simulink model "SIMPLEAC"  (R2020b)
settings: Solver=VariableStepAuto  StartTime=0.0  StopTime=7200  RelTol=1e-3
libraries: simulink x3
settings Model: Creator=99003197  LastModifiedBy=99003181
settings DebuggingCC: ArithmeticOperatorsInVariantConditions=warning
settings SFSimCC: CustomCodeUndefinedFunction=UseInterfaceOnly

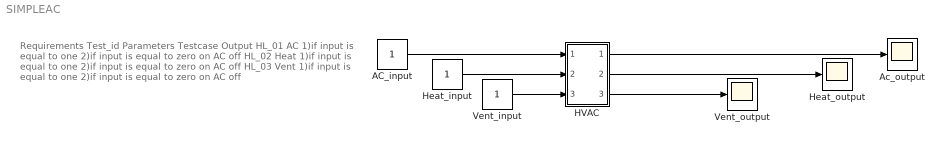
== system SIMPLEAC ==
  note: Requirements
      | Test_id
      | Parameters
      | Testcase
      | Output
      |
      | HL_01
      | AC
      | 1)if input is equal to one
      | 2)if input is equal to zero
      |
      | on
      |
      | AC off
      |
      | HL_02
      | Heat
      | 1)if input is equal to one
      | 2)if input is equal to zero
      | on
      |
      | AC off
      |
      | HL_03
      | Vent
      | 1)if input is equal to one
      | 2)if input is equal to zero
      | on
      |
      | AC off
  AC_input : Constant
  Ac_output : Scope
  HVAC : Subsystem
  Heat_input : Constant
  Heat_output : Scope
  Vent_input : Constant
  Vent_output : Scope
  wires:
  Heat_input/1 -> HVAC/2(Input1)
  AC_input/1 -> HVAC/1(Input)
  HVAC/1(Output) -> Ac_output/1
  Vent_input/1 -> HVAC/3(Input2)
  HVAC/2(Output1) -> Heat_output/1
  HVAC/3(Output2) -> Vent_output/1

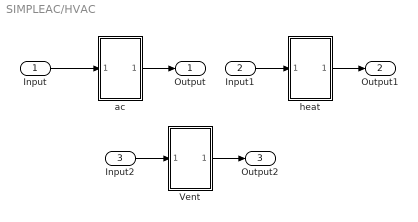
== system SIMPLEAC/HVAC ==
  Input : Inport
  Input1 : Inport  Port=2
  Input2 : Inport  Port=3
  Vent : Subsystem
  ac : Subsystem
  heat : Subsystem
  Output : Outport
  Output1 : Outport  Port=2
  Output2 : Outport  Port=3
  wires:
  Input/1 -> ac/1(Input)
  Input1/1 -> heat/1(Input)
  ac/1(Output) -> Output/1
  heat/1(Output) -> Output1/1
  Input2/1 -> Vent/1(Input)
  Vent/1(Output) -> Output2/1

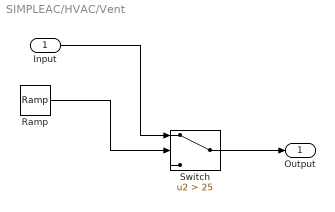
== system SIMPLEAC/HVAC/Vent ==
  Input : Inport
  Ramp : simulink/Sources/Ramp  slope=-0.0069  start=0  InitialOutput=50
  Switch : Switch  Criteria=u2 > Threshold  Threshold=25
  Output : Outport
  wires:
  Ramp/1 -> Switch/2
  Input/1 -> Switch/1
  Switch/1 -> Output/1

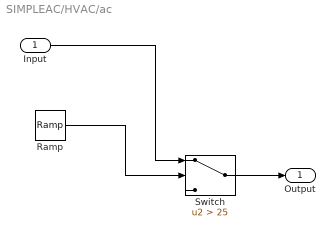
== system SIMPLEAC/HVAC/ac ==
  Input : Inport
  Ramp : simulink/Sources/Ramp  slope=.0069  start=0  InitialOutput=0
  Switch : Switch  Criteria=u2 > Threshold  Threshold=25
  Output : Outport
  wires:
  Input/1 -> Switch/1
  Ramp/1 -> Switch/2
  Switch/1 -> Output/1

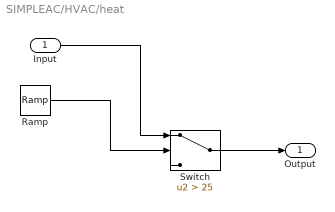
== system SIMPLEAC/HVAC/heat ==
  Input : Inport
  Ramp : simulink/Sources/Ramp  slope=-0.0069  start=0  InitialOutput=50
  Switch : Switch  Criteria=u2 > Threshold  Threshold=25
  Output : Outport
  wires:
  Ramp/1 -> Switch/2
  Input/1 -> Switch/1
  Switch/1 -> Output/1
